simulink model "Problem4"  (R2020b)
settings: Solver=FixedStepDiscrete  StartTime=0.0  StopTime=10.0  FixedStep=Auto  RelTol=1e-3
settings Model: Creator=omkar  LastModifiedBy=omkar

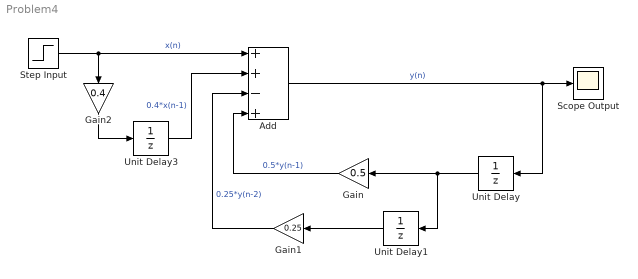
== system Problem4 ==
  Add : Sum  Inputs=++-+
  Gain : Gain  Gain=0.5
  Gain1 : Gain  Gain=0.25
  Gain2 : Gain  Gain=0.4
  Scope Output : Scope
  Step Input : Step  SampleTime=0
  Unit Delay : UnitDelay  SampleTime=-1  HasFrameUpgradeWarning=on
  Unit Delay1 : UnitDelay  SampleTime=-1  HasFrameUpgradeWarning=on
  Unit Delay3 : UnitDelay  SampleTime=-1  HasFrameUpgradeWarning=on
  wires:
  Step Input/1 -> Add/1, Gain2/1  "x(n)"
  Gain2/1 -> Unit Delay3/1
  Unit Delay3/1 -> Add/2  "0.4*x(n-1)"
  Gain/1 -> Add/4  "0.5*y(n-1)"
  Gain1/1 -> Add/3  "0.25*y(n-2)"
  Unit Delay/1 -> Unit Delay1/1, Gain/1
  Unit Delay1/1 -> Gain1/1
  Add/1 -> Unit Delay/1, Scope Output/1  "y(n)"
